simulink subsystem "up_converter"  (R2022b)
settings: Solver=VariableStepAuto  StartTime=0.0  StopTime=10.0  RelTol=1e-3
undefined symbols (not defined in the file or in its folder): rf, S
libraries: simrfV2elements x15, simrfV2sources1 x2, simrfV2_lib x1, simrfV2util1 x1
settings Model: Creator=hessam  LastModifiedBy=hessam

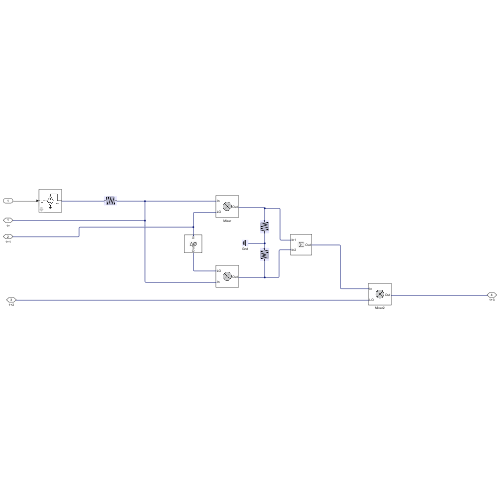
[thumbnail: Simulink's stored preview of the top-level diagram]
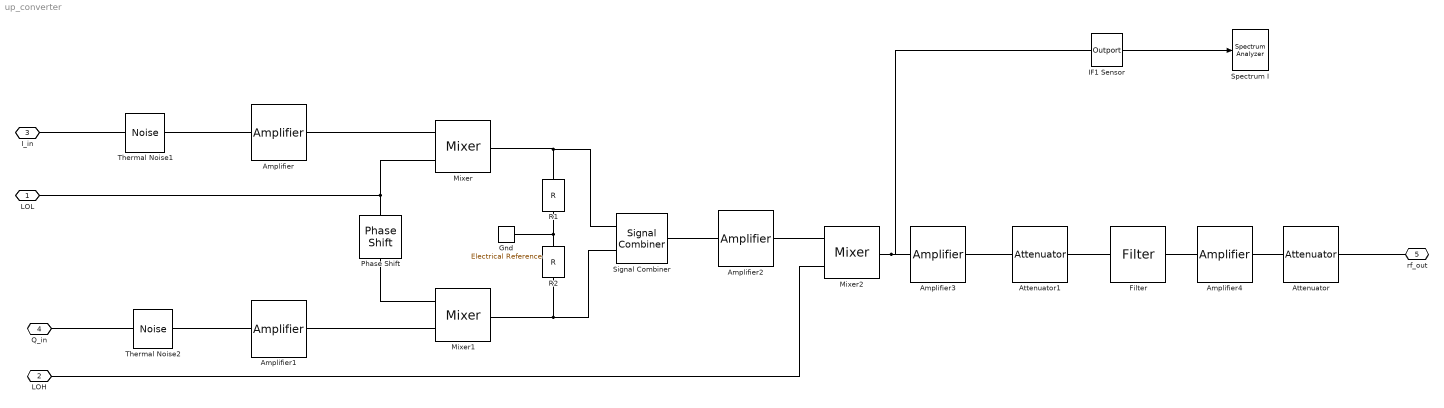
== system up_converter ==
  Amplifier : simrfV2elements/Amplifier  classname=amplifier  DataSource=Data file  File=unitygain.s2p  isNetworkObj=off  Paramtype=S-parameters  Sparam=[0 0;1 0]  SparamFreq=1e9 Hz  SparamZ0=50  isRationalObj=off  Residues=0  Poles=0  DF={0 0; 1 0}  Source_linear_gain=Available power gain  linear_gain=0 dB  AmAmAmPmTable=[-25,5,-1;-10,20,-2;0,27,5;5,28,12]  Zin=50  Zout=50  Source_Poly=Even and odd order  Poly_Coeffs=[0 1]  IPType=Output  IP2=Inf dBm  IP3=inf dBm  P1dB=inf dBm  Psat=inf dBm  Gcomp=inf dBm  InternalGrounding=on  SourceFreq=Extracted from data source  PlotFreq=[1e9:1e6:3e9] Hz  PlotType=X-Y plane  YParam1=S(1,1)  YFormat1=Magnitude (dB)  YParam2=None  YFormat2=Magnitude (dB)  YOption=Linear  XOption=Linear  SparamRepresentation=Time domain (rationalfit)  FitTol=-40  FitOpt=Fit individually  MaxPoles=48  AutoImpulseLength=on  ImpulseLength=1e-10 s  MagModeling=off  AddNoise=on  NoiseType=Noise figure  NoiseDist=White  NF=25  MinNF=0  Gopt=0  RN=0  CarrierFreq=0 Hz  NoiseAutoImpulseLength=on  NoiseImpulseLength=1e-10 s  ConstS21NL=off  OpFreq=1 GHz  SetOpFreqAsMaxS21=off
  Amplifier1 : simrfV2elements/Amplifier  classname=amplifier  DataSource=Data file  File=unitygain.s2p  isNetworkObj=off  Paramtype=S-parameters  Sparam=[0 0;1 0]  SparamFreq=1e9 Hz  SparamZ0=50  isRationalObj=off  Residues=0  Poles=0  DF={0 0; 1 0}  Source_linear_gain=Available power gain  linear_gain=0 dB  AmAmAmPmTable=[-25,5,-1;-10,20,-2;0,27,5;5,28,12]  Zin=50  Zout=50  Source_Poly=Even and odd order  Poly_Coeffs=[0 1]  IPType=Output  IP2=Inf dBm  IP3=Inf dBm  P1dB=inf dBm  Psat=inf dBm  Gcomp=inf dBm  InternalGrounding=on  SourceFreq=Extracted from data source  PlotFreq=[1e9:1e6:3e9] Hz  PlotType=X-Y plane  YParam1=S(1,1)  YFormat1=Magnitude (dB)  YParam2=None  YFormat2=Magnitude (dB)  YOption=Linear  XOption=Linear  SparamRepresentation=Time domain (rationalfit)  FitTol=-40  FitOpt=Fit individually  MaxPoles=48  AutoImpulseLength=on  ImpulseLength=1e-10 s  MagModeling=off  AddNoise=on  NoiseType=Noise figure  NoiseDist=White  NF=25  MinNF=0  Gopt=0  RN=0  CarrierFreq=0 Hz  NoiseAutoImpulseLength=on  NoiseImpulseLength=1e-10 s  ConstS21NL=off  OpFreq=1 GHz  SetOpFreqAsMaxS21=off
  Amplifier2 : simrfV2elements/Amplifier  classname=amplifier  DataSource=Data file  File=unitygain.s2p  isNetworkObj=off  Paramtype=S-parameters  Sparam=[0 0;1 0]  SparamFreq=1e9 Hz  SparamZ0=50  isRationalObj=off  Residues=0  Poles=0  DF={0 0; 1 0}  Source_linear_gain=Available power gain  linear_gain=12 dB  AmAmAmPmTable=[-25,5,-1;-10,20,-2;0,27,5;5,28,12]  Zin=50  Zout=50  Source_Poly=Even and odd order  Poly_Coeffs=[0 1]  IPType=Output  IP2=Inf dBm  IP3=40 dBm  P1dB=inf dBm  Psat=inf dBm  Gcomp=inf dBm  InternalGrounding=on  SourceFreq=Extracted from data source  PlotFreq=[1e9:1e6:3e9] Hz  PlotType=X-Y plane  YParam1=S(1,1)  YFormat1=Magnitude (dB)  YParam2=None  YFormat2=Magnitude (dB)  YOption=Linear  XOption=Linear  SparamRepresentation=Time domain (rationalfit)  FitTol=-40  FitOpt=Fit individually  MaxPoles=48  AutoImpulseLength=on  ImpulseLength=1e-10 s  MagModeling=off  AddNoise=on  NoiseType=Noise figure  NoiseDist=White  NF=15  MinNF=0  Gopt=0  RN=0  CarrierFreq=0 Hz  NoiseAutoImpulseLength=on  NoiseImpulseLength=1e-10 s  ConstS21NL=off  OpFreq=1 GHz  SetOpFreqAsMaxS21=off
  Amplifier3 : simrfV2elements/Amplifier  classname=amplifier  DataSource=Data file  File=unitygain.s2p  isNetworkObj=off  Paramtype=S-parameters  Sparam=[0 0;1 0]  SparamFreq=1e9 Hz  SparamZ0=50  isRationalObj=off  Residues=0  Poles=0  DF={0 0; 1 0}  Source_linear_gain=Available power gain  linear_gain=9 dB  AmAmAmPmTable=[-25,5,-1;-10,20,-2;0,27,5;5,28,12]  Zin=50  Zout=50  Source_Poly=Even and odd order  Poly_Coeffs=[0 1]  IPType=Output  IP2=Inf dBm  IP3=50 dBm  P1dB=inf dBm  Psat=inf dBm  Gcomp=inf dBm  InternalGrounding=on  SourceFreq=Extracted from data source  PlotFreq=[1e9:1e6:3e9] Hz  PlotType=X-Y plane  YParam1=S(1,1)  YFormat1=Magnitude (dB)  YParam2=None  YFormat2=Magnitude (dB)  YOption=Linear  XOption=Linear  SparamRepresentation=Time domain (rationalfit)  FitTol=-40  FitOpt=Fit individually  MaxPoles=48  AutoImpulseLength=on  ImpulseLength=1e-10 s  MagModeling=off  AddNoise=on  NoiseType=Noise figure  NoiseDist=White  NF=15  MinNF=0  Gopt=0  RN=0  CarrierFreq=0 Hz  NoiseAutoImpulseLength=on  NoiseImpulseLength=1e-10 s  ConstS21NL=off  OpFreq=1 GHz  SetOpFreqAsMaxS21=off
  Amplifier4 : simrfV2elements/Amplifier  classname=amplifier  DataSource=Data file  File=unitygain.s2p  isNetworkObj=off  Paramtype=S-parameters  Sparam=[0 0;1 0]  SparamFreq=1e9 Hz  SparamZ0=50  isRationalObj=off  Residues=0  Poles=0  DF={0 0; 1 0}  Source_linear_gain=Available power gain  linear_gain=10 dB  AmAmAmPmTable=[-25,5,-1;-10,20,-2;0,27,5;5,28,12]  Zin=50  Zout=50  Source_Poly=Even and odd order  Poly_Coeffs=[0 1]  IPType=Output  IP2=Inf dBm  IP3=45 dBm  P1dB=inf dBm  Psat=inf dBm  Gcomp=inf dBm  InternalGrounding=on  SourceFreq=Extracted from data source  PlotFreq=[1e9:1e6:3e9] Hz  PlotType=X-Y plane  YParam1=S(1,1)  YFormat1=Magnitude (dB)  YParam2=None  YFormat2=Magnitude (dB)  YOption=Linear  XOption=Linear  SparamRepresentation=Time domain (rationalfit)  FitTol=-40  FitOpt=Fit individually  MaxPoles=48  AutoImpulseLength=on  ImpulseLength=1e-10 s  MagModeling=off  AddNoise=on  NoiseType=Noise figure  NoiseDist=White  NF=25  MinNF=0  Gopt=0  RN=0  CarrierFreq=0 Hz  NoiseAutoImpulseLength=on  NoiseImpulseLength=1e-10 s  ConstS21NL=off  OpFreq=1 GHz  SetOpFreqAsMaxS21=off
  Attenuator : simrfV2elements/Attenuator  classname=attenuator  Att=4  Zin=50  Zout=50  AddNoise=on  InternalGrounding=on
  Attenuator1 : simrfV2elements/Attenuator  classname=attenuator  Att=6  Zin=50  Zout=50  AddNoise=on  InternalGrounding=on
  Filter : simrfV2elements/Filter  classname=filter  DesignMethod=Butterworth  ResponseType=Bandstop  Implementation=LC Tee  ImplementationIdeal=Constant per carrier  ImplementationRational=Transfer function  UseFilterOrder=on  FilterOrder=3  PassFreq_lp=1 GHz  PassFreq_hp=2 GHz  PassFreq_bp=[2 3] GHz  PassFreq_bs=[1 4] GHz  PassAtten=10*log10(2)  StopFreq_lp=2 GHz  StopFreq_hp=1 GHz  StopFreq_bp=[1.5 3.5] GHz  StopFreq_bs=[51 55] GHz  StopAtten=40  Rsrc=50  Rload=50  AutoImpulseLength=on  ImpulseLength=1e-10 s  InternalGrounding=on  PlotFuncLeft=Voltage transfer  PlotLeftForm=Magnitude (dB)  PlotRightOnVT=None  PlotRightNoTD=None  PlotRightNoGD=None  PlotRightNoIR=None  PlotRightNoSR=None  PlotRightForm=Magnitude (dB)  FreqPoints=logspace(0,10,101)  Freq_unit=Hz  TimePoints=linspace(0,1,1e6+1)  Time_unit=s  XaxisScale=Linear  YaxisScale=Linear  needRedraw=0
  Gnd : simrfV2_lib/Elements/Electrical Reference
      settings: InternalSimscapePortConfiguration="{\"Bottom\":[],\"Left\":[{\"id\":\"V\",\"label\":\"\",\"type\":\"foundation.rf.circuitenvelope\"}],\"Right\":[],\"Top\":[]}"
  IF1 Sensor : simrfV2util1/Outport  SensorType=Ideal voltage  OutputFormat=Complex Baseband  CarrierFreq=carriers.OUT Hz  ZL=Inf  InternalGrounding=on  StepSize=-1 s  AutoStep=off
  Mixer : simrfV2elements/Mixer  classname=mixer  Source_linear_gain=Available power gain  linear_gain=0 dB  Zin=50  Zout=50  ZLO=inf  Source_Poly=Even and odd order  Poly_Coeffs=0  IPType=Output  IP2=Inf dBm  IP3=35 dBm  P1dB=Inf dBm  Psat=Inf dBm  Gcomp=Inf dBm  NF=25  InternalGrounding=on
  Mixer1 : simrfV2elements/Mixer  classname=mixer  Source_linear_gain=Available power gain  linear_gain=0 dB  Zin=50  Zout=50  ZLO=50  Source_Poly=Even and odd order  Poly_Coeffs=0  IPType=Output  IP2=Inf dBm  IP3=35 dBm  P1dB=Inf dBm  Psat=Inf dBm  Gcomp=Inf dBm  NF=25  InternalGrounding=on
  Mixer2 : simrfV2elements/Mixer  classname=mixer  Source_linear_gain=Available power gain  linear_gain=-6 dB  Zin=50  Zout=50  ZLO=inf  Source_Poly=Even and odd order  Poly_Coeffs=0  IPType=Output  IP2=Inf dBm  IP3=40 dBm  P1dB=Inf dBm  Psat=Inf dBm  Gcomp=Inf dBm  NF=15  InternalGrounding=on
  Phase Shift : simrfV2elements/Phase Shift  PhaseShift=90 deg  InternalGrounding=on
  R1 : simrfV2elements/R  classname=resistor  Resistance=50 Ohm  AddNoise=on
  R2 : simrfV2elements/R  classname=resistor  Resistance=50 Ohm  AddNoise=on
  Signal Combiner : simrfV2elements/Signal Combiner  classname=signal_sum_mask  InternalGrounding=on
  Spectrum I : SpectrumAnalyzer
  Thermal Noise1 : simrfV2sources1/Noise  SimulinkInputSignalType=Ideal voltage  NoiseType=White  NoisePSD=4*rf.physconst('Boltzmann')*290*50  CarrierFreq=0 Hz  AutoImpulseLength=on  ImpulseLength=1e-10 s  InternalGrounding=off
  Thermal Noise2 : simrfV2sources1/Noise  SimulinkInputSignalType=Ideal voltage  NoiseType=White  NoisePSD=4*rf.physconst('Boltzmann')*290*50  CarrierFreq=0 Hz  AutoImpulseLength=on  ImpulseLength=1e-10 s  InternalGrounding=off
  LOL : PMIOPort  Side=Left
  LOH : PMIOPort  Port=2  Side=Left
  I_in : PMIOPort  Port=3  Side=Left
  Q_in : PMIOPort  Port=4  Side=Left
  rf_out : PMIOPort  Port=5  Side=Left
  wires:
  IF1 Sensor/1 -> Spectrum I/1
  connections:
  Mixer2/RConn1 -- Amplifier3/LConn1 -- IF1 Sensor/LConn1
  Phase Shift/LConn1 -- Mixer/LConn2 -- LOL/RConn1
  R1/RConn1 -- R2/LConn1 -- Gnd/LConn1
  Mixer1/RConn1 -- R2/RConn1 -- Signal Combiner/LConn2
  R1/LConn1 -- Mixer/RConn1 -- Signal Combiner/LConn1
  rf_out/RConn1 -- Attenuator/RConn1
  Q_in/RConn1 -- Thermal Noise2/RConn1
  I_in/RConn1 -- Thermal Noise1/RConn1
  Attenuator1/RConn1 -- Filter/LConn1
  Amplifier4/RConn1 -- Attenuator/LConn1
  Filter/RConn1 -- Amplifier4/LConn1
  Amplifier2/RConn1 -- Mixer2/LConn1
  Amplifier2/LConn1 -- Signal Combiner/RConn1
  Amplifier1/LConn1 -- Thermal Noise2/LConn1
  Amplifier1/RConn1 -- Mixer1/LConn1
  Amplifier/RConn1 -- Mixer/LConn1
  Amplifier/LConn1 -- Thermal Noise1/LConn1
  LOH/RConn1 -- Mixer2/LConn2
  Phase Shift/RConn1 -- Mixer1/LConn2
  Amplifier3/RConn1 -- Attenuator1/LConn1
